simulink model "untitled"  (R2021a)
settings: Solver=FixedStepAuto  StartTime=0.0  StopTime=30  FixedStep=0.001  RelTol=1e-3
values from neighbouring files (symbols this model uses):
  kp = 0.5*ku    (= 0.688)    [Q5.m]
  Td = 0.3*Tdu    (= 0.285)    [Q5.m]
  Ti = 3.3*Tiu    (= 2.145)    [Q5.m]
libraries: simulink x2
settings Model: Creator=M.M  LastModifiedBy=M.M

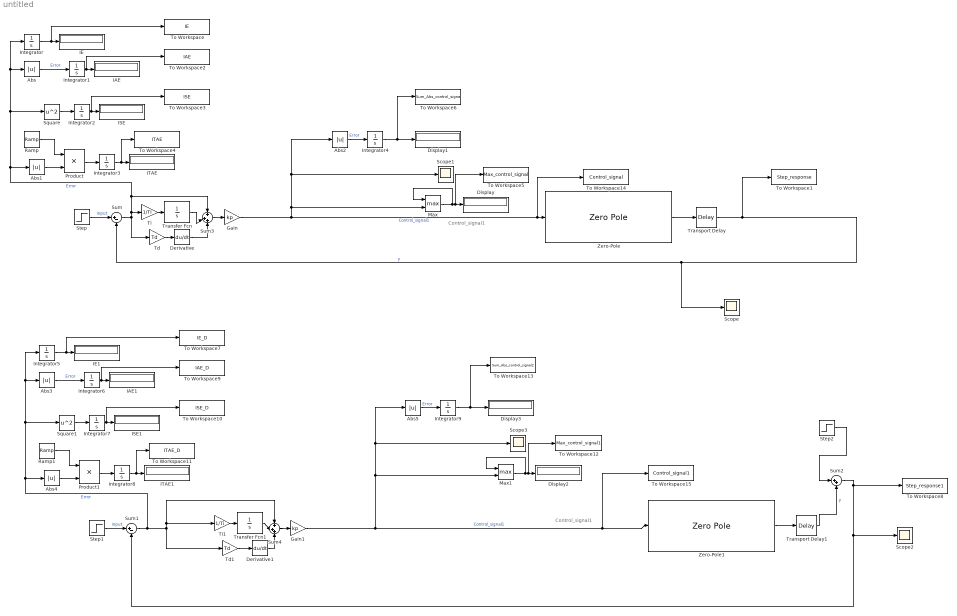
== system untitled ==
  note: Control_signal1
  note: Control_signal1
  Abs{,1..5} (6 alike) : Abs
  Derivative : Derivative
  Derivative1 : Derivative
  Display{,1..3} (4 alike) : Display
  Gain : Gain  Gain=kp
  Gain1 : Gain  Gain=kp
  IAE : Display
  IAE1 : Display
  IE : Display
  IE1 : Display
  ISE : Display
  ISE1 : Display
  ITAE : Display
  ITAE1 : Display
  Integrator{,1..9} (10 alike) : Integrator
  Max : MinMax  Function=max  Inputs=2
  Max1 : MinMax  Function=max  Inputs=2
  Product : Product
  Product1 : Product
  Ramp : simulink/Sources/Ramp  slope=1  start=0  InitialOutput=0
  Ramp1 : simulink/Sources/Ramp  slope=1  start=0  InitialOutput=0
  Scope{,1..3} (4 alike) : Scope
  Square : Math  Operator=square  SaturateOnIntegerOverflow=on
  Square1 : Math  Operator=square  SaturateOnIntegerOverflow=on
  Step : Step  Time=0  SampleTime=0
  Step1 : Step  Time=0  SampleTime=0
  Step2 : Step  Time=15  After=0.5  SampleTime=0
  Sum : Sum  Inputs=|+-
  Sum1 : Sum  Inputs=|+-
  Sum2 : Sum  Inputs=|++
  Sum3 : Sum  Inputs=+|++
  Sum4 : Sum  Inputs=+|++
  Td : Gain  Gain=Td
  Td1 : Gain  Gain=Td
  Ti : Gain  Gain=1/Ti
  Ti1 : Gain  Gain=1/Ti
  To Workspace : ToWorkspace  VariableName=IE  SaveFormat=Timeseries  SampleTime=-1
  To Workspace1 : ToWorkspace  VariableName=Step_response  SaveFormat=Timeseries  SampleTime=-1
  To Workspace10 : ToWorkspace  VariableName=ISE_D  SaveFormat=Timeseries  SampleTime=-1
  To Workspace11 : ToWorkspace  VariableName=ITAE_D  SaveFormat=Timeseries  SampleTime=-1
  To Workspace12 : ToWorkspace  VariableName=Max_control_signal1  SaveFormat=Timeseries  SampleTime=-1
  To Workspace13 : ToWorkspace  VariableName=Sum_Abs_control_signal2  SaveFormat=Timeseries  SampleTime=-1
  To Workspace14 : ToWorkspace  VariableName=Control_signal  SaveFormat=Timeseries  SampleTime=-1
  To Workspace15 : ToWorkspace  VariableName=Control_signal1  SaveFormat=Timeseries  SampleTime=-1
  To Workspace2 : ToWorkspace  VariableName=IAE  SaveFormat=Timeseries  SampleTime=-1
  To Workspace3 : ToWorkspace  VariableName=ISE  SaveFormat=Timeseries  SampleTime=-1
  To Workspace4 : ToWorkspace  VariableName=ITAE  SaveFormat=Timeseries  SampleTime=-1
  To Workspace5 : ToWorkspace  VariableName=Max_control_signal  SaveFormat=Timeseries  SampleTime=-1
  To Workspace6 : ToWorkspace  VariableName=Sum_Abs_control_signal  SaveFormat=Timeseries  SampleTime=-1
  To Workspace7 : ToWorkspace  VariableName=IE_D  SaveFormat=Timeseries  SampleTime=-1
  To Workspace8 : ToWorkspace  VariableName=Step_response1  SaveFormat=Timeseries  SampleTime=-1
  To Workspace9 : ToWorkspace  VariableName=IAE_D  SaveFormat=Timeseries  SampleTime=-1
  Transfer Fcn : TransferFcn  Denominator=[1 0]
  Transfer Fcn1 : TransferFcn  Denominator=[1 0]
  Transport Delay : TransportDelay  DelayTime=0.633
  Transport Delay1 : TransportDelay  DelayTime=0.633
  Zero-Pole : ZeroPole  Zeros=[]  Poles=[-1 -5 -25 -125]  Gain=[2*5*25*125]
  Zero-Pole1 : ZeroPole  Zeros=[]  Poles=[-1 -5 -25 -125]  Gain=[2*5*25*125]
  wires:
  Step/1 -> Sum/1  "input"
  Zero-Pole/1 -> Transport Delay/1
  Transport Delay/1 -> To Workspace1/1, Sum/2, Scope/1  "y"
  Sum/1 -> Td/1, Ti/1, Abs1/1, Abs/1, Integrator/1, Square/1, Sum3/1  "Error"
  Max/1 -> Max/1, To Workspace5/1, Display/1
  Integrator/1 -> To Workspace/1, IE/1
  Abs/1 -> Integrator1/1  "Error"
  Integrator1/1 -> To Workspace2/1, IAE/1
  Integrator2/1 -> To Workspace3/1, ISE/1
  Square/1 -> Integrator2/1
  Abs1/1 -> Product/2
  Ramp/1 -> Product/1
  Product/1 -> Integrator3/1
  Integrator3/1 -> To Workspace4/1, ITAE/1
  Abs2/1 -> Integrator4/1  "Error"
  Integrator4/1 -> To Workspace6/1, Display1/1
  Step1/1 -> Sum1/1  "input"
  Transport Delay1/1 -> Sum2/2  "y"
  Zero-Pole1/1 -> Transport Delay1/1
  Integrator9/1 -> To Workspace13/1, Display3/1
  Ramp1/1 -> Product1/1
  Integrator8/1 -> To Workspace11/1, ITAE1/1
  Abs5/1 -> Integrator9/1  "Error"
  Max1/1 -> Max1/1, To Workspace12/1, Display2/1
  Integrator7/1 -> To Workspace10/1, ISE1/1
  Square1/1 -> Integrator7/1
  Product1/1 -> Integrator8/1
  Integrator5/1 -> To Workspace7/1, IE1/1
  Abs3/1 -> Integrator6/1  "Error"
  Integrator6/1 -> To Workspace9/1, IAE1/1
  Abs4/1 -> Product1/2
  Step2/1 -> Sum2/1
  Sum2/1 -> To Workspace8/1, Scope2/1, Sum1/2
  Derivative/1 -> Sum3/3
  Td/1 -> Derivative/1
  Transfer Fcn/1 -> Sum3/2
  Ti/1 -> Transfer Fcn/1
  Transfer Fcn1/1 -> Sum4/2
  Td1/1 -> Derivative1/1
  Sum4/1 -> Gain1/1
  Sum1/1 -> Td1/1, Ti1/1, Sum4/1, Abs4/1, Abs3/1, Integrator5/1, Square1/1  "Error"
  Derivative1/1 -> Sum4/3
  Ti1/1 -> Transfer Fcn1/1
  Sum3/1 -> Gain/1
  Gain/1 -> To Workspace14/1, Zero-Pole/1, Abs2/1, Scope1/1, Max/2  "Control_signal1"
  Gain1/1 -> Abs5/1, Scope3/1, Max1/2, To Workspace15/1, Zero-Pole1/1  "Control_signal1"
